simulink model "SuperStepSemantics"  (R2020a)
settings: Solver=FixedStepDiscrete  StartTime=0.0  StopTime=50.0  FixedStep=1  RelTol=1e-3
libraries: simulink x1
settings Model: Creator=ashok  LastModifiedBy=ashok
settings RTWCC: Description=Create Visual C/C++ Solution File for Simulink Coder  TemplateMakefile=RTW.MSVCBuild

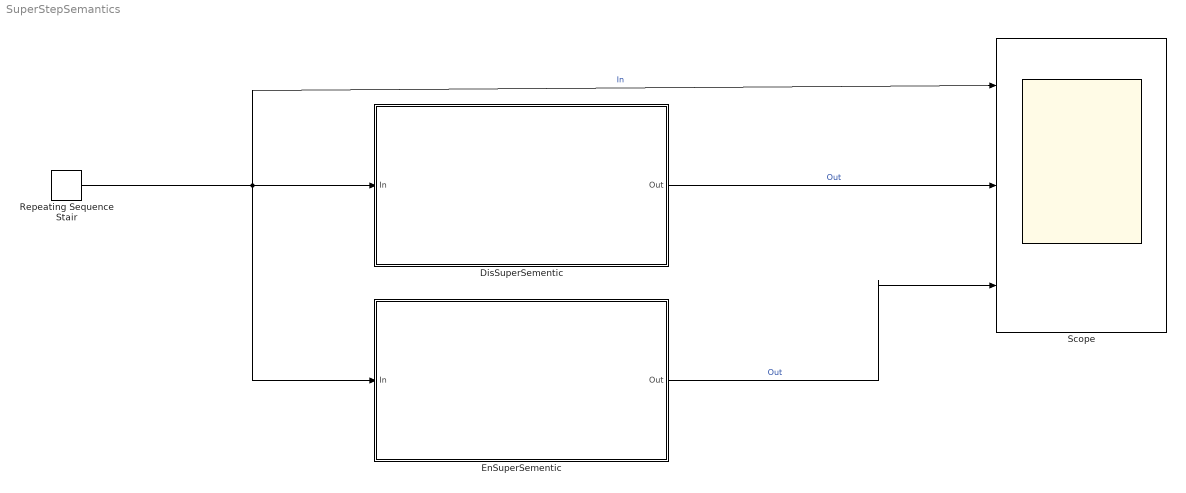
== system SuperStepSemantics ==
  DisSuperSementic : Stateflow chart  TreatAsAtomicUnit=on
  EnSuperSementic : Stateflow chart  TreatAsAtomicUnit=on
  Repeating Sequence Stair : simulink/Sources/Repeating Sequence Stair  OutValues=In  tsamp=-1  OutMin=[]  OutMax=[]  OutDataTypeStr=double  OutputDataTypeScalingMode=double  OutDataType=fixdt(0,8)  ConRadixGroup=Best Precision: Vector-wise  OutScaling=2^-12
  Scope : Scope  NumInputPorts=3
  wires:
  DisSuperSementic/1(Out) -> Scope/2  "Out"
  Repeating Sequence Stair/1 -> EnSuperSementic/1(In), Scope/1, DisSuperSementic/1(In)  "In"
  EnSuperSementic/1(Out) -> Scope/3  "Out"

== stateflow chart SuperStepSemantics/EnSuperSementic ==
  settings: enableNonTerminalStates=1
  state STATE_A
    entry:
    Out = 1;
  state STATE_B
    entry:
    Out = 2;
  state STATE_C
    entry:
    Out = 3;
  (default) -> STATE_A
  STATE_A -> STATE_B : [In > 5]
  STATE_B -> STATE_A [order 1] : [In <= 5]
  STATE_B -> STATE_C [order 2] : [In > 10]
  STATE_C -> STATE_B : [In <= 10]
  data: In input; Out output

== stateflow chart SuperStepSemantics/DisSuperSementic ==
  state STATE_A
    entry:
    Out = 1;
  state STATE_B
    entry:
    Out = 2;
  state STATE_C
    entry:
    Out = 3;
  (default) -> STATE_A
  STATE_A -> STATE_B : [In > 5]
  STATE_B -> STATE_A [order 1] : [In <= 5]
  STATE_B -> STATE_C [order 2] : [In > 10]
  STATE_C -> STATE_B : [In <= 10]
  data: In input; Out output
